simulink model "Subsystem"  (R2017b)
settings: Solver=FixedStepDiscrete  StartTime=0.0  StopTime=10.0  FixedStep=0.200000  RelTol=1e-3
settings Model: Creator=hbourbou  LastModifiedBy=hbourbou
settings DataIOCC: SaveFormat=StructureWithTime
settings OptimizationCC: LifeSpan=inf
settings DebuggingCC: SFExecutionAtInitializationDiag=none
settings HardwareCC: ProdBitPerSizeT=32  ProdBitPerPtrDiffT=32  ProdWordSize=32  ProdHWDeviceType=Specified
settings CodeAppCC: StateflowObjectComments=on

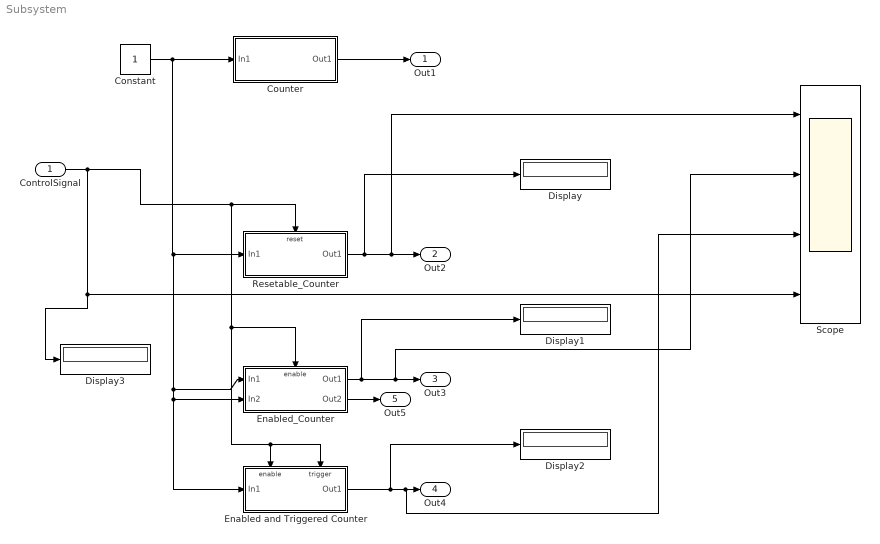
== system Subsystem ==
  ControlSignal : Inport
  Constant : Constant
  Counter : Subsystem
  Display{,1..3} (4 alike) : Display
  Enabled and Triggered Counter : Subsystem  TreatAsAtomicUnit=on
  Enabled_Counter : Subsystem  TreatAsAtomicUnit=on
  Resetable_Counter : Subsystem
  Scope : Scope  NumInputPorts=4
  Out1 : Outport
  Out2 : Outport  Port=2
  Out3 : Outport  Port=3
  Out4 : Outport  Port=4
  Out5 : Outport  Port=5
  wires:
  Counter/1(Out1) -> Out1/1
  Constant/1 -> Enabled and Triggered Counter/1(In1), Enabled_Counter/2(In2), Enabled_Counter/1(In1), Resetable_Counter/1(In1), Counter/1(In1)
  Resetable_Counter/1(Out1) -> Display/1, Scope/1, Out2/1
  Enabled_Counter/1(Out1) -> Display1/1, Scope/2, Out3/1
  ControlSignal/1 -> Display3/1, Scope/4, Enabled and Triggered Counter/Trigger, Enabled and Triggered Counter/Enable, Enabled_Counter/Enable, Resetable_Counter/Reset
  Enabled and Triggered Counter/1(Out1) -> Display2/1, Scope/3, Out4/1
  Enabled_Counter/2(Out2) -> Out5/1

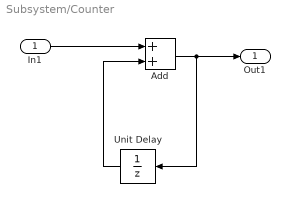
== system Subsystem/Counter ==
  In1 : Inport
  Add : Sum
  Unit Delay : UnitDelay  SampleTime=-1
  Out1 : Outport
  wires:
  In1/1 -> Add/1
  Add/1 -> Unit Delay/1, Out1/1
  Unit Delay/1 -> Add/2

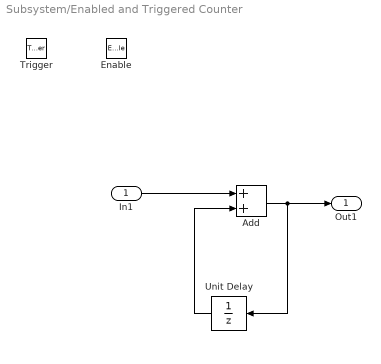
== system Subsystem/Enabled and Triggered Counter ==
  In1 : Inport
  Enable : EnablePort  StatesWhenEnabling=reset
  Trigger : TriggerPort  VariantControl=(inherit)
  Add : Sum
  Unit Delay : UnitDelay  SampleTime=-1
  Out1 : Outport
  wires:
  In1/1 -> Add/1
  Add/1 -> Unit Delay/1, Out1/1
  Unit Delay/1 -> Add/2

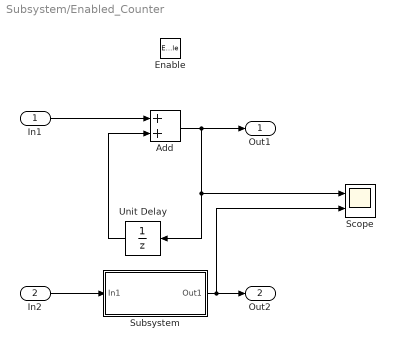
== system Subsystem/Enabled_Counter ==
  In1 : Inport
  In2 : Inport  Port=2
  Enable : EnablePort
  Add : Sum
  Scope : Scope  NumInputPorts=2
  Subsystem : Subsystem  TreatAsAtomicUnit=on
  Unit Delay : UnitDelay  SampleTime=-1
  Out1 : Outport  OutputWhenDisabled=reset  InitialOutput=0.2
  Out2 : Outport  Port=2
  wires:
  In1/1 -> Add/1
  Unit Delay/1 -> Add/2
  Subsystem/1(Out1) -> Scope/2, Out2/1
  In2/1 -> Subsystem/1(In1)
  Add/1 -> Scope/1, Unit Delay/1, Out1/1

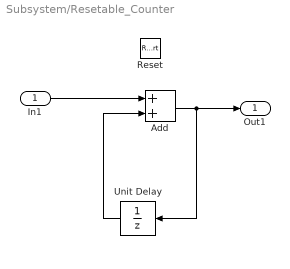
== system Subsystem/Resetable_Counter ==
  In1 : Inport
  Reset : ResetPort  DisableCoverage=on
  Add : Sum
  Unit Delay : UnitDelay  SampleTime=-1
  Out1 : Outport
  wires:
  In1/1 -> Add/1
  Add/1 -> Unit Delay/1, Out1/1
  Unit Delay/1 -> Add/2

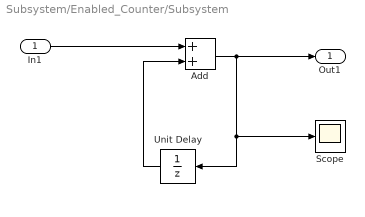
== system Subsystem/Enabled_Counter/Subsystem ==
  In1 : Inport
  Add : Sum
  Scope : Scope
  Unit Delay : UnitDelay  SampleTime=-1
  Out1 : Outport
  wires:
  In1/1 -> Add/1
  Unit Delay/1 -> Add/2
  Add/1 -> Scope/1, Unit Delay/1, Out1/1
